simulink model "Ex3"  (R2023b)
settings: Solver=FixedStepDiscrete  StartTime=0.0  StopTime=inf  RelTol=1e-3
PreLoadFcn:
  | Apass = 0.005; % dB
  | Astop = 80; % dB
  | Fstop = .101;
  | M = 7;
  | F = [.1 Fstop];
  | A = [convertmagunits(Apass,'db','linear','pass') convertmagunits(Astop,'db','linear','stop')];
  | [h,g]=ifir(M,'low',F,A);
undefined symbols (not defined in the file): designMultirateFIR
libraries: dspmlti4 x4
CloseFcn:
  | clear Apass Astop Fstop M F A h g
settings Model: Creator=Fartash  LastModifiedBy=Fartash
settings SolverCC: AlgebraicLoopSolver=TrustRegion  AutoInsertRateTranBlk=on  MaxZcPerStep=1
settings DataIOCC: LimitDataPoints=on  SaveOutput=off  SignalLogging=off  SaveTime=off
settings OptimizationCC: ReuseModelBlockBuffer=off  LifeSpan=inf  SimCompilerOptimization=on
settings DebuggingCC: AlgebraicLoopMsg=error  SingleTaskRateTransMsg=error  IntegerOverflowMsg=none  ParameterPrecisionLossMsg=none  UnconnectedInputMsg=warning  UnconnectedOutputMsg=warning  UnconnectedLineMsg=warning  AllowSymbolicDim=off  SubsystemReferenceDiagnosticForUnitTest=warning  SFUnexpectedBacktrackingDiag=warning  SFNoUnconditionalDefaultTransitionDiag=warning  SFExecutionAtInitializationDiag=none  IntegerSaturationMsg=none  ArithmeticOperatorsInVariantConditions=warning
settings ModelReferenceCC: EnableRefExpFcnMdlSchedulingChecks=on
settings SFSimCC: SimCtrlC=off  SimUseLocalCustomCode=off  CustomCodeUndefinedFunction=UseInterfaceOnly
settings RTWCC: RTWUseLocalCustomCode=off  DLArmComputeVersion=19.05
settings CodeAppCC: StateflowObjectComments=on
settings GRTTargetCC: TargetLangStandard=C89/C90 (ANSI)
settings ConfigComp: CovMetricSettings=dw  CovSaveCumulativeToWorkspaceVar=on  CovSaveSingleToWorkspaceVar=on  CovExternalEMLEnable=off  CovSFcnEnable=off

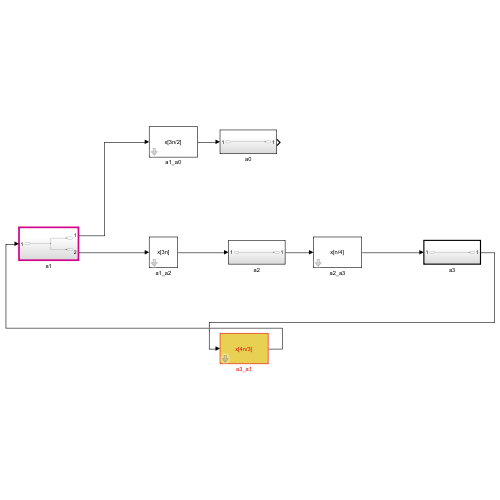
[thumbnail: Simulink's stored preview of the top-level diagram]
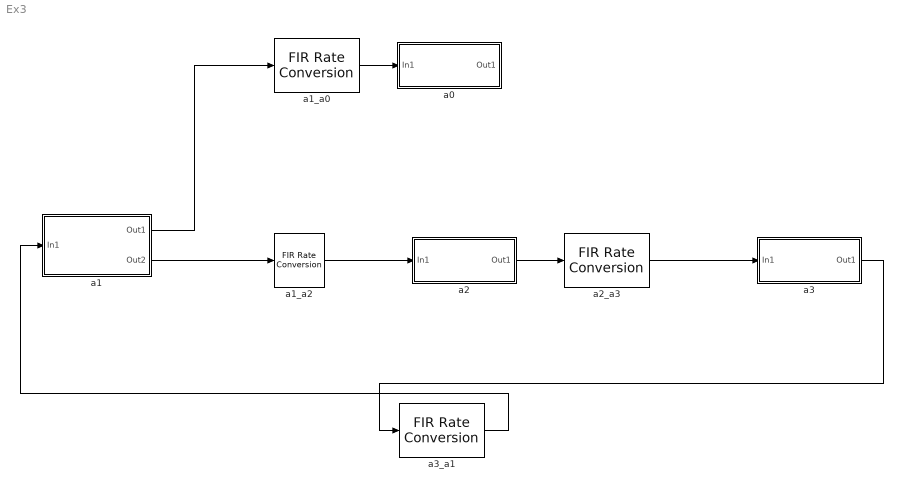
== system Ex3 ==
  a0 : Subsystem
  a1 : Subsystem  TreatAsAtomicUnit=on
  a1_a0 : dspmlti4/FIR Rate Conversion  FilterSource=Auto  L=2  h=designMultirateFIR(3,2)  M=3  FilterObject=FRC  rateMode=Allow multirate processing  AllowArbitraryInputLength=off  roundingMode=Floor  overflowMode=off  firstCoeffDataTypeStr=Inherit: Same word length as input  firstCoeffMin=[]  firstCoeffMax=[]  firstCoeffLastDataTypeStr=Inherit: Same word length as input  outputDataTypeStr=Inherit: Same as accumulator  outputMin=[]  outputMax=[]  outputLastDataTypeStr=Inherit: Same as accumulator
  a1_a2 : dspmlti4/FIR Rate Conversion  FilterSource=Auto  L=1  h=designMultirateFIR(3,2)  M=3  FilterObject=FRC  rateMode=Allow multirate processing  AllowArbitraryInputLength=off  roundingMode=Floor  overflowMode=off  firstCoeffDataTypeStr=Inherit: Same word length as input  firstCoeffMin=[]  firstCoeffMax=[]  firstCoeffLastDataTypeStr=Inherit: Same word length as input  outputDataTypeStr=Inherit: Same as accumulator  outputMin=[]  outputMax=[]  outputLastDataTypeStr=Inherit: Same as accumulator
      settings: LockScale=on
  a2 : Subsystem
  a2_a3 : dspmlti4/FIR Rate Conversion  FilterSource=Auto  L=4  h=designMultirateFIR(3,2)  M=1  FilterObject=FRC  rateMode=Allow multirate processing  AllowArbitraryInputLength=off  roundingMode=Floor  overflowMode=off  firstCoeffDataTypeStr=Inherit: Same word length as input  firstCoeffMin=[]  firstCoeffMax=[]  firstCoeffLastDataTypeStr=Inherit: Same word length as input  outputDataTypeStr=Inherit: Same as accumulator  outputMin=[]  outputMax=[]  outputLastDataTypeStr=Inherit: Same as accumulator
  a3 : Subsystem  TreatAsAtomicUnit=on
  a3_a1 : dspmlti4/FIR Rate Conversion  FilterSource=Auto  L=3  h=designMultirateFIR(3,2)  M=4  FilterObject=FRC  rateMode=Allow multirate processing  AllowArbitraryInputLength=off  roundingMode=Floor  overflowMode=off  firstCoeffDataTypeStr=Inherit: Same word length as input  firstCoeffMin=[]  firstCoeffMax=[]  firstCoeffLastDataTypeStr=Inherit: Same word length as input  outputDataTypeStr=Inherit: Same as accumulator  outputMin=[]  outputMax=[]  outputLastDataTypeStr=Inherit: Same as accumulator
  wires:
  a1_a2/1 -> a2/1(In1)
  a2/1(Out1) -> a2_a3/1
  a2_a3/1 -> a3/1(In1)
  a3_a1/1 -> a1/1(In1)
  a3/1(Out1) -> a3_a1/1
  a1_a0/1 -> a0/1(In1)
  a1/1(Out1) -> a1_a0/1
  a1/2(Out2) -> a1_a2/1

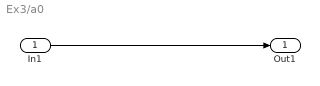
== system Ex3/a0 ==
  In1 : Inport
  Out1 : Outport
  wires:
  In1/1 -> Out1/1

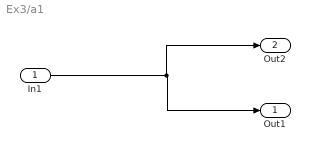
== system Ex3/a1 ==
  In1 : Inport
  Out1 : Outport
  Out2 : Outport  Port=2
  wires:
  In1/1 -> Out2/1, Out1/1

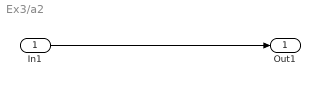
== system Ex3/a2 ==
  In1 : Inport
  Out1 : Outport
  wires:
  In1/1 -> Out1/1

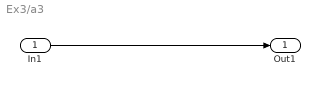
== system Ex3/a3 ==
  In1 : Inport
  Out1 : Outport
  wires:
  In1/1 -> Out1/1
